simulink model "avlAerodynamics_th"  (R2018b)
settings: Solver=VariableStepAuto  StartTime=0.0  StopTime=0  RelTol=1e-3
values from neighbouring files (symbols this model uses):
  ailDefl_deg = 0    [avlAerodynamics_ts.m]
  dynPress = 1    [avlAerodynamics_ts.m]
  elevDefl_deg = 0    [avlAerodynamics_ts.m]
  flpDefl_deg = 0    [avlAerodynamics_ts.m]
  refArea = 1    [avlAerodynamics_ts.m]
  rudDefl_deg = 0    [avlAerodynamics_ts.m]
  uAppBdy = [5 0 -1]    [avlAerodynamics_ts.m]
undefined symbols (not defined in the file or in its folder): avlAerodynamics, CLtotTbl
libraries: alphaBeta_ul x1
settings Model: Creator=mcobb  LastModifiedBy=mcobb

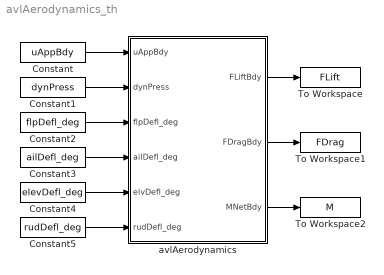
== system avlAerodynamics_th ==
  Constant : Constant  Value=uAppBdy
  Constant1 : Constant  Value=dynPress
  Constant2 : Constant  Value=flpDefl_deg
  Constant3 : Constant  Value=ailDefl_deg
  Constant4 : Constant  Value=elevDefl_deg
  Constant5 : Constant  Value=rudDefl_deg
  To Workspace : ToWorkspace  VariableName=FLift  SaveFormat=Timeseries  SampleTime=-1
  To Workspace1 : ToWorkspace  VariableName=FDrag  SaveFormat=Timeseries  SampleTime=-1
  To Workspace2 : ToWorkspace  VariableName=M  SaveFormat=Timeseries  SampleTime=-1
  avlAerodynamics : Subsystem  AncestorBlock=avlAerodynamics/avlAerodynamics  mask{CLTable=CLtotTbl, CDTable=CLtotTbl, CMxTable=CLtotTbl, CMyTable=CLtotTbl, CMzTable=CLtotTbl, SRef=1, BRef=1, CRef=1}
      mask prompts: CLTable "CL lookup table object"; CDTable "CD lookup table object"; CMxTable "CMx lookup table object"; CMyTable "CMy lookup table object"; CMzTable "CMz lookup table object"; SRef "Ref area (AVL Sref)"; BRef "Roll & Yaw Moment Reference Length (AVL Bref)"; CRef "Pitch Moment Reference Length (AVL Cref)"
      mask DialogControl Container4 Prompt: Reference Areas
  wires:
  Constant/1 -> avlAerodynamics/1(uAppBdy)
  Constant4/1 -> avlAerodynamics/5(elvDefl_deg)
  Constant3/1 -> avlAerodynamics/4(ailDefl_deg)
  Constant2/1 -> avlAerodynamics/3(flpDefl_deg)
  Constant1/1 -> avlAerodynamics/2(dynPress)
  avlAerodynamics/3(MNetBdy) -> To Workspace2/1
  avlAerodynamics/2(FDragBdy) -> To Workspace1/1
  avlAerodynamics/1(FLiftBdy) -> To Workspace/1
  Constant5/1 -> avlAerodynamics/6(rudDefl_deg)

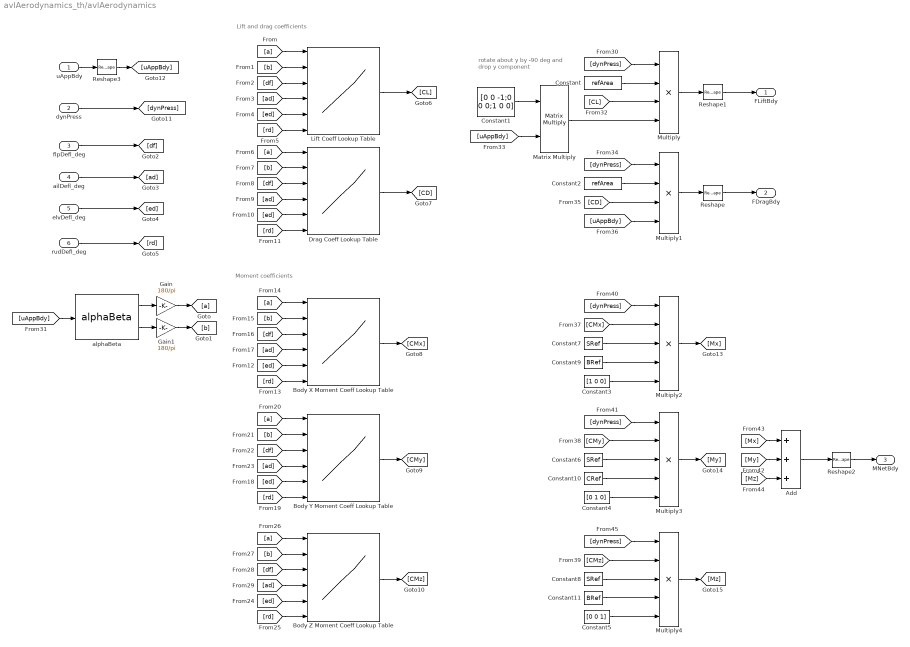
== system avlAerodynamics_th/avlAerodynamics ==
  note: Lift and drag coefficients
  note: Moment coefficients
  note: rotate about y by -90 deg
      | and drop y component
  uAppBdy : Inport
  dynPress : Inport  Port=2
  flpDefl_deg : Inport  Port=3
  ailDefl_deg : Inport  Port=4
  elvDefl_deg : Inport  Port=5
  rudDefl_deg : Inport  Port=6
  Add : Sum  Inputs=+++
  Body X Moment Coeff Lookup Table : Lookup_n-D  NumberOfTableDimensions=6  DataSpecification=Lookup table object  LookupTableObject=CMxTable  BreakpointsForDimension3=[5, 7]  Table=reshape(repmat([4 5 6;16 19 20;10 18 23],1,2),[3,3,2])  InternalRulePriority=Speed  RndMeth=Simplest  InputSameDT=on
  Body Y Moment Coeff Lookup Table : Lookup_n-D  NumberOfTableDimensions=6  DataSpecification=Lookup table object  LookupTableObject=CMyTable  BreakpointsForDimension3=[5, 7]  Table=reshape(repmat([4 5 6;16 19 20;10 18 23],1,2),[3,3,2])  InternalRulePriority=Speed  RndMeth=Simplest  InputSameDT=on
  Body Z Moment Coeff Lookup Table : Lookup_n-D  NumberOfTableDimensions=6  DataSpecification=Lookup table object  LookupTableObject=CMzTable  BreakpointsForDimension3=[5, 7]  Table=reshape(repmat([4 5 6;16 19 20;10 18 23],1,2),[3,3,2])  InternalRulePriority=Speed  RndMeth=Simplest  InputSameDT=on
  Constant : Constant  Value=refArea
  Constant1 : Constant  Value=[0 0 -1;0 0 0;1 0 0]
  Constant10 : Constant  Value=CRef
  Constant11 : Constant  Value=BRef
  Constant2 : Constant  Value=refArea
  Constant3 : Constant  Value=[1 0 0]
  Constant4 : Constant  Value=[0 1 0]
  Constant5 : Constant  Value=[0 0 1]
  Constant6 : Constant  Value=SRef
  Constant7 : Constant  Value=SRef
  Constant8 : Constant  Value=SRef
  Constant9 : Constant  Value=BRef
  Drag Coeff Lookup Table : Lookup_n-D  NumberOfTableDimensions=6  DataSpecification=Lookup table object  LookupTableObject=CDTable  BreakpointsForDimension3=[5, 7]  Table=reshape(repmat([4 5 6;16 19 20;10 18 23],1,2),[3,3,2])  InternalRulePriority=Speed  RndMeth=Simplest  InputSameDT=on
  Gain : Gain  Gain=180/pi
  Gain1 : Gain  Gain=180/pi
  Lift Coeff Lookup Table : Lookup_n-D  NumberOfTableDimensions=6  DataSpecification=Lookup table object  LookupTableObject=CLTable  BreakpointsForDimension3=[5, 7]  Table=reshape(repmat([4 5 6;16 19 20;10 18 23],1,2),[3,3,2])  InternalRulePriority=Speed  RndMeth=Simplest  InputSameDT=on
  Matrix Multiply : Product  Multiplication=Matrix(*)
  Multiply : Product  Inputs=4
  Multiply1 : Product  Inputs=4
  Multiply2 : Product  Inputs=5
  Multiply3 : Product  Inputs=5
  Multiply4 : Product  Inputs=5
  Reshape{,1..3} (4 alike) : Reshape  OutputDimensionality=Column vector (2-D)
  alphaBeta : alphaBeta_ul/alphaBeta  SystemSampleTime=-1
  FLiftBdy : Outport
  FDragBdy : Outport  Port=2
  MNetBdy : Outport  Port=3
  wires:
  Constant11/1 -> Multiply4/4
  Constant10/1 -> Multiply3/4
  [dynPress] -> Multiply2/1
  Constant9/1 -> Multiply2/4
  [dynPress] -> Multiply4/1
  [dynPress] -> Multiply3/1
  Constant5/1 -> Multiply4/5
  Constant4/1 -> Multiply3/5
  Constant3/1 -> Multiply2/5
  Constant8/1 -> Multiply4/3
  Constant6/1 -> Multiply3/3
  Constant7/1 -> Multiply2/3
  Reshape3/1 -> [uAppBdy]
  Reshape2/1 -> MNetBdy/1
  Add/1 -> Reshape2/1
  [Mz] -> Add/3
  [Mx] -> Add/1
  [My] -> Add/2
  Multiply4/1 -> [Mz]
  [CMz] -> Multiply4/2
  [CMy] -> Multiply3/2
  Multiply3/1 -> [My]
  Multiply2/1 -> [Mx]
  [CMx] -> Multiply2/2
  Reshape/1 -> FDragBdy/1
  Reshape1/1 -> FLiftBdy/1
  Multiply1/1 -> Reshape/1
  Multiply/1 -> Reshape1/1
  [uAppBdy] -> Multiply1/4
  [dynPress] -> Multiply1/1
  Constant2/1 -> Multiply1/2
  [CD] -> Multiply1/3
  [uAppBdy] -> Matrix Multiply/2
  Constant1/1 -> Matrix Multiply/1
  Matrix Multiply/1 -> Multiply/4
  [CL] -> Multiply/3
  Constant/1 -> Multiply/2
  [dynPress] -> Multiply/1
  [uAppBdy] -> alphaBeta/1
  dynPress/1 -> [dynPress]
  Gain1/1 -> [b]
  Gain/1 -> [a]
  alphaBeta/2 -> Gain1/1
  alphaBeta/1 -> Gain/1
  Body Y Moment Coeff Lookup Table/1 -> [CMy]
  Body X Moment Coeff Lookup Table/1 -> [CMx]
  Drag Coeff Lookup Table/1 -> [CD]
  [rd] -> Body Z Moment Coeff Lookup Table/6
  [ed] -> Body Z Moment Coeff Lookup Table/5
  [ad] -> Body Z Moment Coeff Lookup Table/4
  [df] -> Body Z Moment Coeff Lookup Table/3
  [a] -> Body Z Moment Coeff Lookup Table/1
  [b] -> Body Z Moment Coeff Lookup Table/2
  [b] -> Body Y Moment Coeff Lookup Table/2
  [a] -> Body Y Moment Coeff Lookup Table/1
  [df] -> Body Y Moment Coeff Lookup Table/3
  [ad] -> Body Y Moment Coeff Lookup Table/4
  [ed] -> Body Y Moment Coeff Lookup Table/5
  [rd] -> Body Y Moment Coeff Lookup Table/6
  [rd] -> Body X Moment Coeff Lookup Table/6
  [ed] -> Body X Moment Coeff Lookup Table/5
  [ad] -> Body X Moment Coeff Lookup Table/4
  [df] -> Body X Moment Coeff Lookup Table/3
  [a] -> Body X Moment Coeff Lookup Table/1
  [b] -> Body X Moment Coeff Lookup Table/2
  [b] -> Drag Coeff Lookup Table/2
  [a] -> Drag Coeff Lookup Table/1
  [df] -> Drag Coeff Lookup Table/3
  [ad] -> Drag Coeff Lookup Table/4
  [ed] -> Drag Coeff Lookup Table/5
  [rd] -> Drag Coeff Lookup Table/6
  Lift Coeff Lookup Table/1 -> [CL]
  [rd] -> Lift Coeff Lookup Table/6
  [ed] -> Lift Coeff Lookup Table/5
  [ad] -> Lift Coeff Lookup Table/4
  [df] -> Lift Coeff Lookup Table/3
  [a] -> Lift Coeff Lookup Table/1
  [b] -> Lift Coeff Lookup Table/2
  rudDefl_deg/1 -> [rd]
  elvDefl_deg/1 -> [ed]
  ailDefl_deg/1 -> [ad]
  flpDefl_deg/1 -> [df]
  uAppBdy/1 -> Reshape3/1
  Body Z Moment Coeff Lookup Table/1 -> [CMz]
